simulink model "c6711dskDIPswitch"  (Simulink 6.0)
settings: Solver=FixedStepDiscrete  StartTime=0.0  StopTime=inf  RelTol=1e-3
libraries: c6711dsklib x4, dspsigops x4, c6000tgtpreflib x1
settings Model: Creator=zgalijas  LastModifiedBy=thartley  RTWExpressionDepthLimit=1  ProdHWDeviceType=TI C6000
settings DataIOCC: LimitDataPoints=off  SaveOutput=off  SaveTime=off  SignalLoggingName=sigsOut
settings OptimizationCC: InlineParams=on  InlineInvariantSignals=off  EnforceIntegerDowncast=off
settings DebuggingCC: CheckExecutionContextPreStartOutputMsg=on  CheckExecutionContextRuntimeOutputMsg=on  SolverPrmCheckMsg=none
settings HardwareCC: ProdBitPerLong=40  ProdEndianess=LittleEndian  ProdHWDeviceType=TI C6000
settings ModelReferenceCC: UpdateModelReferenceTargets=IfOutOfDate
settings RTWCC: SystemTargetFile=ti_c6000.tlc  TemplateMakefile=ti_c6000.tmf  ProcessScript=ti_c6000_make_rtw_hook
settings CodeAppCC: PrefixModelToSubsysFcnNames=off
settings STFCustomTargetCC: TargetFcnLib=ansi_tfl_tmw.mat  MatFileLogging=on  LifeSpan=inf  SystemTargetFile=ti_c6000.tlc  ActivateCallback=c6000_callback('ActivateCallback',hSrc,hDlg);
settings GRTTargetCC: ModelReferenceCompliant=off  LifeSpan=inf
settings CustomProperty: DataType=RTWOptions_EnumType_S__A_matlab_toolbox_rtw_targets_tic6000_tic6000_ti_c6000_BoardType  Value=C6711DSK
settings EnumStrPairs: String=C6416DSK
settings SFSimCC: SFSimApplyToAllLibs=on  SFSimBuildMode=Incremental

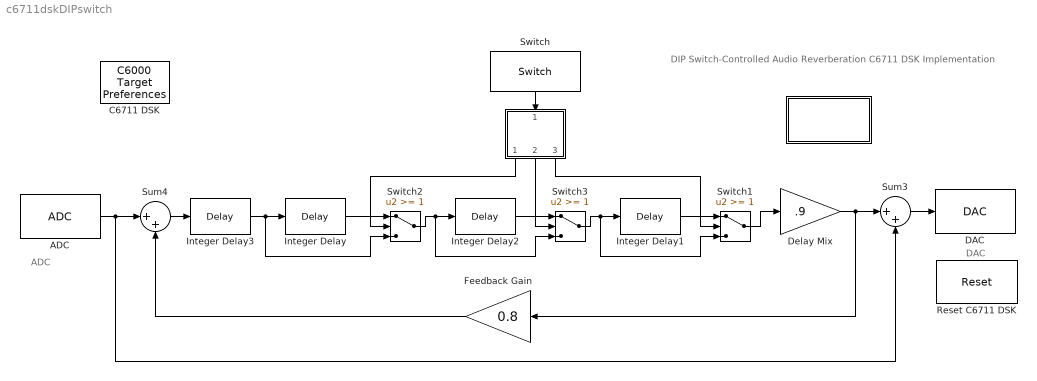
== system c6711dskDIPswitch ==
  note: DIP Switch-Controlled Audio Reverberation
      | C6711 DSK Implementation
  note: ADC
  note: DAC
  " " : Subsystem
      mask Display: disp('Info')
  "  " : Subsystem  Orientation=down
  ADC : c6711dsklib/ADC  ADCsource=Mic In  MicGain=on  OutputDataType=Double  Scaling=Normalize  SourceGain=4.5  FrameSize=64
  C6711 DSK : c6000tgtpreflib/C6000 Target Preferences
  DAC : c6711dsklib/DAC  Scaling=Normalize  DacAtten=0.0  OverflowMode=Saturate
  Delay Mix : Gain  Gain=.9  SaturateOnIntegerOverflow=on
  Feedback Gain : Gain  Orientation=left  Gain=0.8  SaturateOnIntegerOverflow=on
  Integer Delay{,1..3} (4 alike) : dspsigops/Delay  delay=450  ic=0  reset_popup=None
  Reset C6711 DSK : c6711dsklib/Reset
  Sum3 : Sum  Inputs=|++  SaturateOnIntegerOverflow=on  InputSameDT=on
  Sum4 : Sum  Inputs=|++  SaturateOnIntegerOverflow=on  InputSameDT=on
  Switch : c6711dsklib/Switch  Orientation=down  sw1=off  sw2=off  sw3=off  dType=Boolean  Ts=64/8000
  Switch1 : Switch  Threshold=1  ZeroCross=off  InputSameDT=on
  Switch2 : Switch  Threshold=1  ZeroCross=off  InputSameDT=on
  Switch3 : Switch  Threshold=1  ZeroCross=off  InputSameDT=on
  wires:
  Sum3/1 -> DAC/1
  ADC/1 -> Sum3/2, Sum4/1
  Feedback Gain/1 -> Sum4/2
  Delay Mix/1 -> Feedback Gain/1, Sum3/1
  Switch1/1 -> Delay Mix/1
  Integer Delay1/1 -> Switch1/1
  Integer Delay/1 -> Switch2/1
  Switch2/1 -> Integer Delay2/1, Switch3/3
  "  "/1(SW1) -> Switch2/2
  Sum4/1 -> Integer Delay3/1
  Integer Delay3/1 -> Integer Delay/1, Switch2/3
  Integer Delay2/1 -> Switch3/1
  Switch3/1 -> Integer Delay1/1, Switch1/3
  "  "/2(SW2) -> Switch3/2
  "  "/3(SW3) -> Switch1/2
  Switch/1 -> "  "/1("   ")

== system c6711dskDIPswitch/  ==
  note: DIP Switch-Controlled Audio Reverberation
      | C6711 DSK Implementation
      |
      | This simulation of audio reverberation demonstrates the use of the C6711 DSK DIP Switch block.
      | This block reads the status of user-controlled DIP switches (USER_SW1, USER_SW2,
      | USER_SW3) on the c6711 DSK board. Each DIP switch controls a corresponding delay block.

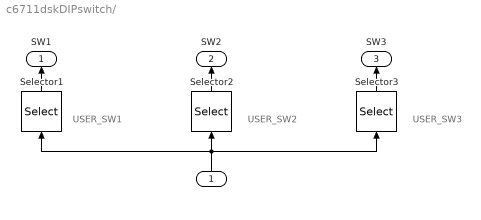
== system c6711dskDIPswitch/   ==
  note: USER_SW1
  note: USER_SW2
  note: USER_SW3
  "   " : Inport  Orientation=up
  Selector1 : Selector  Orientation=up  InputPortWidth=3
  Selector2 : Selector  Orientation=up  Elements=2  InputPortWidth=3
  Selector3 : Selector  Orientation=up  Elements=3  InputPortWidth=3
  SW1 : Outport  Orientation=up
  SW2 : Outport  Orientation=up  Port=2
  SW3 : Outport  Orientation=up  Port=3
  wires:
  "   "/1 -> Selector2/1, Selector3/1, Selector1/1
  Selector1/1 -> SW1/1
  Selector2/1 -> SW2/1
  Selector3/1 -> SW3/1
